simulink model "Transmission_Line"  (R2023b)
settings: Solver=VariableStepAuto  StartTime=0.0  StopTime=1  RelTol=1e-3
libraries: spsVoltageMeasurementLib x2, spsACVoltageSourceLib x1, spsParallelRLCBranchLib x1, spsPiSectionLineLib x1, spsSeriesRLCBranchLib x1, spsSeriesRLCLoadLib x1, sps_lib x1
settings Model: Creator=HP  LastModifiedBy=HP

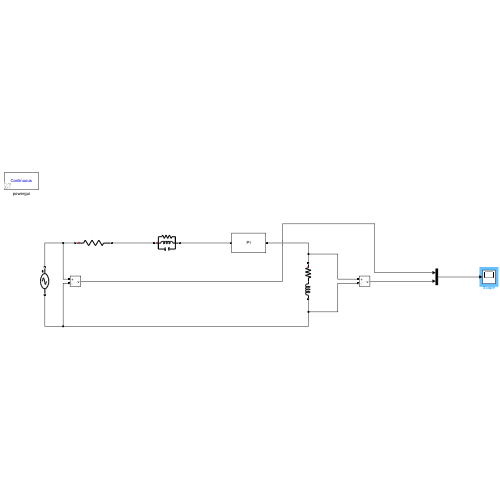
[thumbnail: Simulink's stored preview of the top-level diagram]
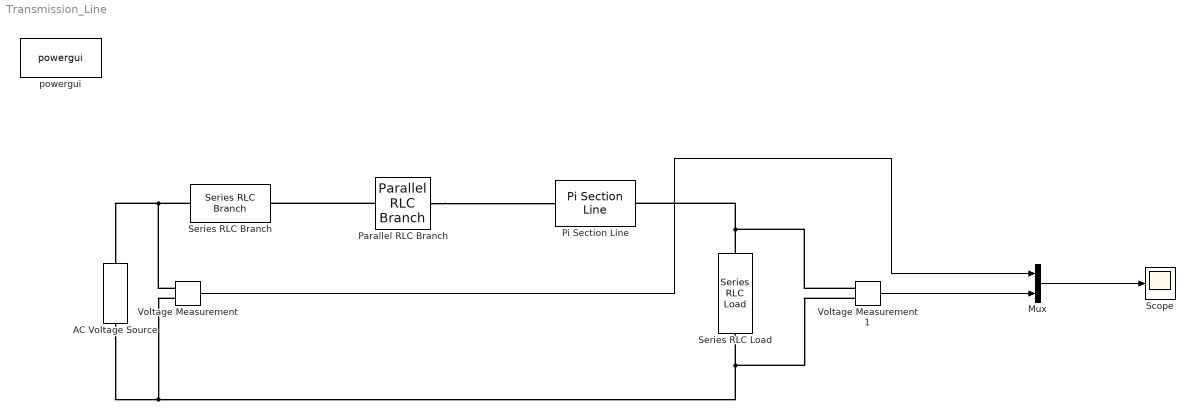
== system Transmission_Line ==
  AC Voltage Source : spsACVoltageSourceLib/AC Voltage Source  Amplitude=424.4e3*sqrt(2)  Phase=0  Frequency=50  SampleTime=0  Measurements=None  BusType=swing  Pref=10e3  Qref=0  Qmin=-inf  Qmax=+inf
  Mux : Mux  Inputs=2
  Parallel RLC Branch : spsParallelRLCBranchLib/Parallel RLC Branch  LConnTagsString=a  RConnTagsString=__new0  BranchType=RLC  Resistance=180  Inductance=26.525e-3  SetiL0=off  InitialCurrent=0  Capacitance=117.84e-6  Setx0=off  InitialVoltage=0  Measurements=None
  Pi Section Line : spsPiSectionLineLib/Pi Section Line  LConnTagsString=1  RConnTagsString=1  Phases=1  PiSections=1  Length=300  Frequency=60  Resistance=0.011  Inductance=0.8674e-3  Capacitance=13.41e-9  SpecifyConductance=off  Conductance=0  Measurements=None  Measurements2=None
      settings: LibrarySourceBlock=sps_lib/Power Grid Elements/Pi Section Line
  Scope : Scope
  Series RLC Branch : spsSeriesRLCBranchLib/Series RLC Branch  LConnTagsString=__new0  RConnTagsString=__new0  BranchType=R  Resistance=2  Inductance=1e-3  SetiL0=off  InitialCurrent=0  Capacitance=1e-6  Setx0=off  InitialVoltage=0  Measurements=None
  Series RLC Load : spsSeriesRLCLoadLib/Series RLC Load  LConnTagsString=a  RConnTagsString=__new0  NominalVoltage=424.4e3  NominalFrequency=50  ActivePower=110e6/300  InductivePower=110e6  CapacitivePower=0  Setx0=on  InitialVoltage=0  SetiL0=on  InitialCurrent=0  Measurements=None  LoadType=constant Z
  Voltage Measurement : spsVoltageMeasurementLib/Voltage Measurement  PhasorSimulation=off  OutputType=Complex  PSBequivalent=0
  Voltage Measurement1 : spsVoltageMeasurementLib/Voltage Measurement  PhasorSimulation=off  OutputType=Complex  PSBequivalent=0
  powergui : sps_lib/powergui  Priority=1  SimulationMode=Continuous  SampleTime=50e-6  frequency=60  Iterations=50  frequencyindice=50  Pbase=100e6  ErrMax=1e-4  UnitsV=kV  UnitsW=MW  buscounter=0  FunctionMessages=off  echomessages=off  EnableUseOfTLC=off  CurrentSourceSwitches=off  DisableSnubberDevices=off  DisableRonSwitches=off  DisableVfSwitches=off  DisplayEquations=off  AutomaticDiscreteSolvers=off  SolverType=Tustin/Backward Euler (TBE)  Interpol=off  ExternalGateDelay=off  methode=off  Ts=100  x0status=blocks  SPID=on  SwTol=0  HookPort=off  NonlinearTolerance=1e-4  nMaxIteration=100  ContinueOnMaxIteration=off  RestoreLinks=warning  ResistiveCurrentMeasurement=off  Frange=[0:2:500]  Ylog=off  Xlog=on  ShowGrid=off  save=off  variable=ZData  structure=0  ZoomFFT=off  StartTime=0.0  cycles=1  DisplayStyle=1  fundamental=60  FreqAxis=off  MaxFrequency=1000  frequencyindicesteady=1  RmsSteady=1  display=off
  wires:
  Voltage Measurement1/1 -> Mux/2
  Voltage Measurement/1 -> Mux/1
  Mux/1 -> Scope/1
  connections:
  Series RLC Branch/LConn1 -- Voltage Measurement/LConn1 -- AC Voltage Source/RConn1
  Parallel RLC Branch/LConn1 -- Series RLC Branch/RConn1
  Parallel RLC Branch/RConn1 -- Pi Section Line/LConn1
  Series RLC Load/LConn1 -- Voltage Measurement1/LConn1 -- Pi Section Line/RConn1
  AC Voltage Source/LConn1 -- Voltage Measurement1/LConn2 -- Series RLC Load/RConn1 -- Voltage Measurement/LConn2
